simulink model "StateError"  (R2017b)
settings: Solver=FixedStepAuto  StartTime=0.0  StopTime=10.0  FixedStep=0.08  RelTol=1e-3
settings Model: Creator=hbourbou  LastModifiedBy=hbourbou

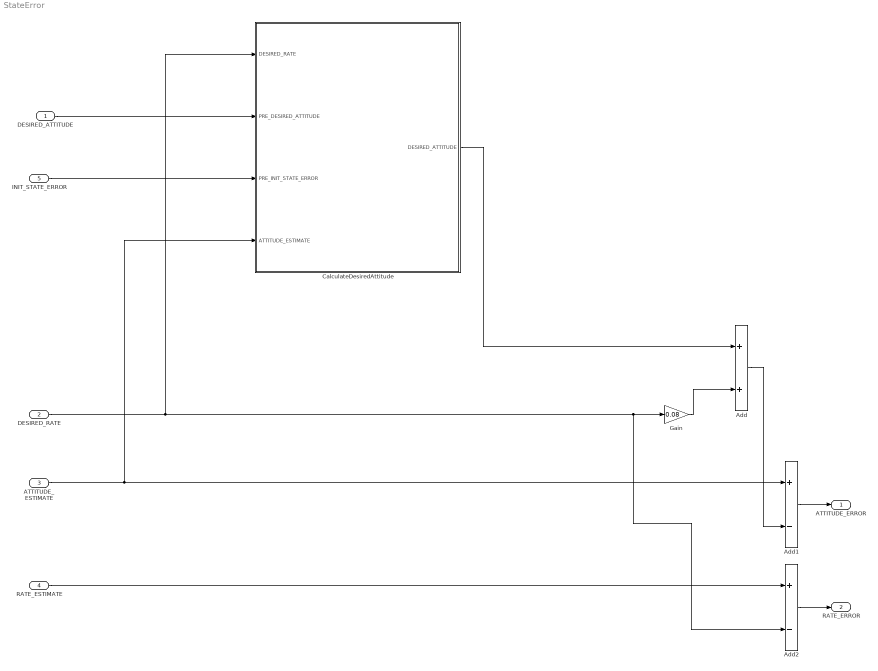
== system StateError ==
  DESIRED_ATTITUDE : Inport  PortDimensions=3
  DESIRED_RATE : Inport  Port=2  PortDimensions=3
  ATTITUDE_ESTIMATE : Inport  Port=3  PortDimensions=3
  RATE_ESTIMATE : Inport  Port=4  PortDimensions=3
  INIT_STATE_ERROR : Inport  Port=5
  Add : Sum
  Add1 : Sum  Inputs=+-
  Add2 : Sum  Inputs=+-
  CalculateDesiredAttitude : Subsystem
  Gain : Gain  Gain=0.08
  ATTITUDE_ERROR : Outport
  RATE_ERROR : Outport  Port=2
  wires:
  RATE_ESTIMATE/1 -> Add2/1
  Add/1 -> Add1/2
  Gain/1 -> Add/2
  Add1/1 -> ATTITUDE_ERROR/1
  CalculateDesiredAttitude/1(DESIRED_ATTITUDE) -> Add/1
  Add2/1 -> RATE_ERROR/1
  ATTITUDE_ESTIMATE/1 -> CalculateDesiredAttitude/4(ATTITUDE_ESTIMATE), Add1/1
  INIT_STATE_ERROR/1 -> CalculateDesiredAttitude/3(PRE_INIT_STATE_ERROR)
  DESIRED_RATE/1 -> CalculateDesiredAttitude/1(DESIRED_RATE), Add2/2, Gain/1
  DESIRED_ATTITUDE/1 -> CalculateDesiredAttitude/2(PRE_DESIRED_ATTITUDE)

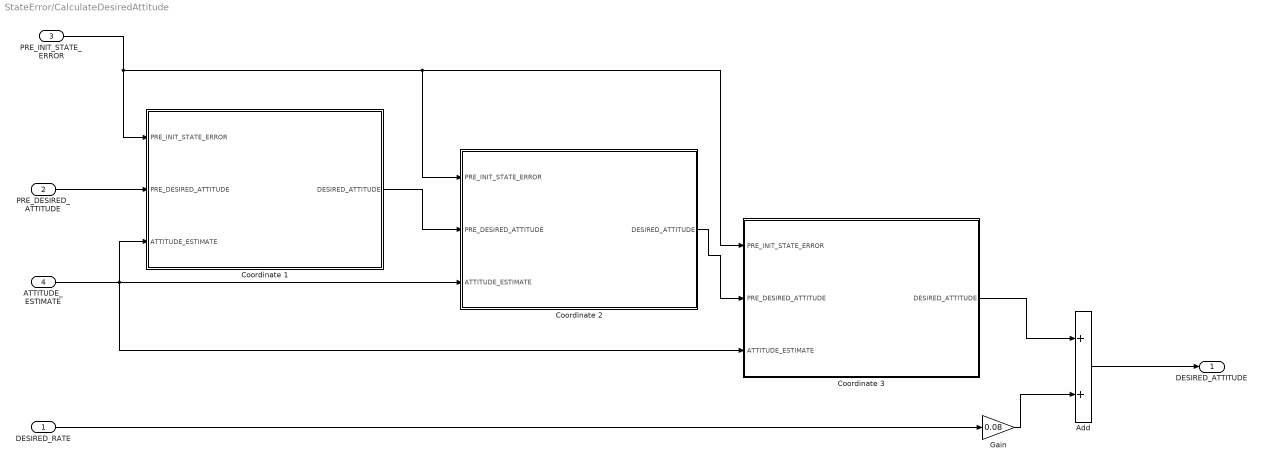
== system StateError/CalculateDesiredAttitude ==
  DESIRED_RATE : Inport  PortDimensions=3
  PRE_DESIRED_ATTITUDE : Inport  Port=2  PortDimensions=3
  PRE_INIT_STATE_ERROR : Inport  Port=3  OutDataTypeStr=boolean  PortDimensions=3
  ATTITUDE_ESTIMATE : Inport  Port=4  PortDimensions=3
  Add : Sum
  Coordinate 1 : Subsystem
  Coordinate 2 : Subsystem
  Coordinate 3 : Subsystem
  Gain : Gain  Gain=0.08
  DESIRED_ATTITUDE : Outport
  wires:
  PRE_INIT_STATE_ERROR/1 -> Coordinate 3/1(PRE_INIT_STATE_ERROR), Coordinate 2/1(PRE_INIT_STATE_ERROR), Coordinate 1/1(PRE_INIT_STATE_ERROR)
  PRE_DESIRED_ATTITUDE/1 -> Coordinate 1/2(PRE_DESIRED_ATTITUDE)
  ATTITUDE_ESTIMATE/1 -> Coordinate 2/3(ATTITUDE_ESTIMATE), Coordinate 3/3(ATTITUDE_ESTIMATE), Coordinate 1/3(ATTITUDE_ESTIMATE)
  Add/1 -> DESIRED_ATTITUDE/1
  Coordinate 3/1(DESIRED_ATTITUDE) -> Add/1
  Coordinate 1/1(DESIRED_ATTITUDE) -> Coordinate 2/2(PRE_DESIRED_ATTITUDE)
  DESIRED_RATE/1 -> Gain/1
  Gain/1 -> Add/2
  Coordinate 2/1(DESIRED_ATTITUDE) -> Coordinate 3/2(PRE_DESIRED_ATTITUDE)

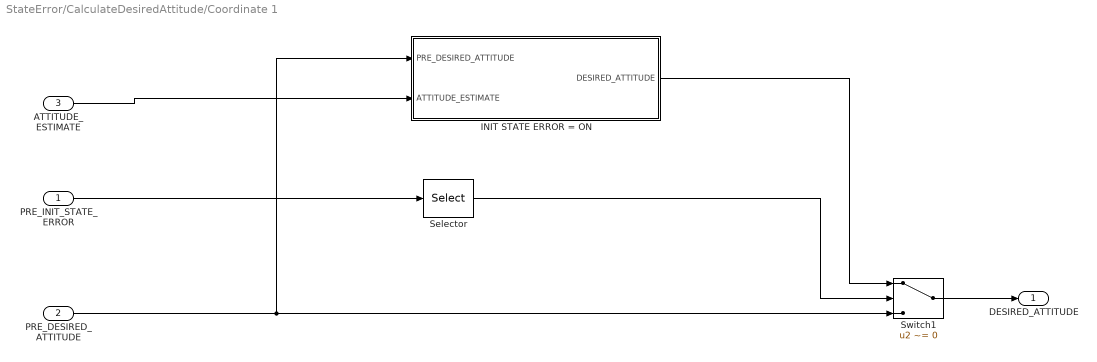
== system StateError/CalculateDesiredAttitude/Coordinate 1 ==
  PRE_INIT_STATE_ERROR : Inport
  PRE_DESIRED_ATTITUDE : Inport  Port=2
  ATTITUDE_ESTIMATE : Inport  Port=3
  INIT STATE ERROR = ON : Subsystem  TreatAsAtomicUnit=on
  Selector : Selector  InputPortWidth=3  IndexOptions=Index vector (dialog)  Indices=[1]  OutputSizes=1
  Switch1 : Switch  Criteria=u2 ~= 0
  DESIRED_ATTITUDE : Outport
  wires:
  PRE_INIT_STATE_ERROR/1 -> Selector/1
  Switch1/1 -> DESIRED_ATTITUDE/1
  INIT STATE ERROR = ON/1(DESIRED_ATTITUDE) -> Switch1/1
  PRE_DESIRED_ATTITUDE/1 -> INIT STATE ERROR = ON/1(PRE_DESIRED_ATTITUDE), Switch1/3
  ATTITUDE_ESTIMATE/1 -> INIT STATE ERROR = ON/2(ATTITUDE_ESTIMATE)
  Selector/1 -> Switch1/2

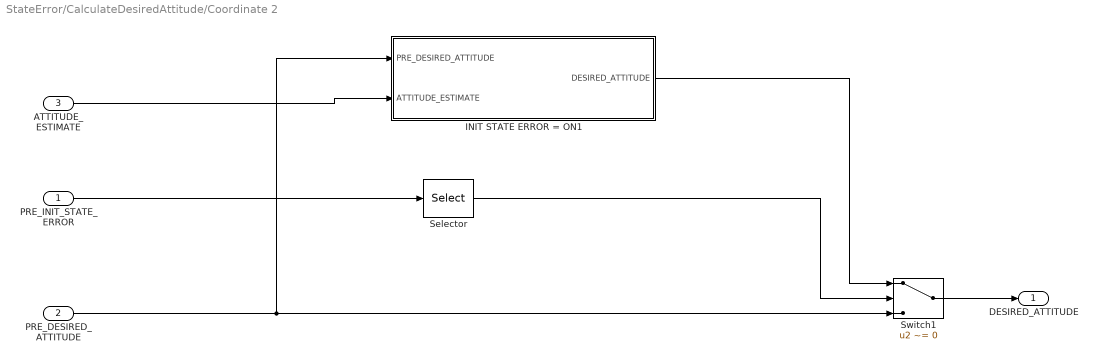
== system StateError/CalculateDesiredAttitude/Coordinate 2 ==
  PRE_INIT_STATE_ERROR : Inport
  PRE_DESIRED_ATTITUDE : Inport  Port=2
  ATTITUDE_ESTIMATE : Inport  Port=3
  INIT STATE ERROR = ON1 : Subsystem  TreatAsAtomicUnit=on
  Selector : Selector  InputPortWidth=3  IndexOptions=Index vector (dialog)  Indices=2  OutputSizes=1
  Switch1 : Switch  Criteria=u2 ~= 0
  DESIRED_ATTITUDE : Outport
  wires:
  PRE_INIT_STATE_ERROR/1 -> Selector/1
  Switch1/1 -> DESIRED_ATTITUDE/1
  INIT STATE ERROR = ON1/1(DESIRED_ATTITUDE) -> Switch1/1
  PRE_DESIRED_ATTITUDE/1 -> INIT STATE ERROR = ON1/1(PRE_DESIRED_ATTITUDE), Switch1/3
  ATTITUDE_ESTIMATE/1 -> INIT STATE ERROR = ON1/2(ATTITUDE_ESTIMATE)
  Selector/1 -> Switch1/2

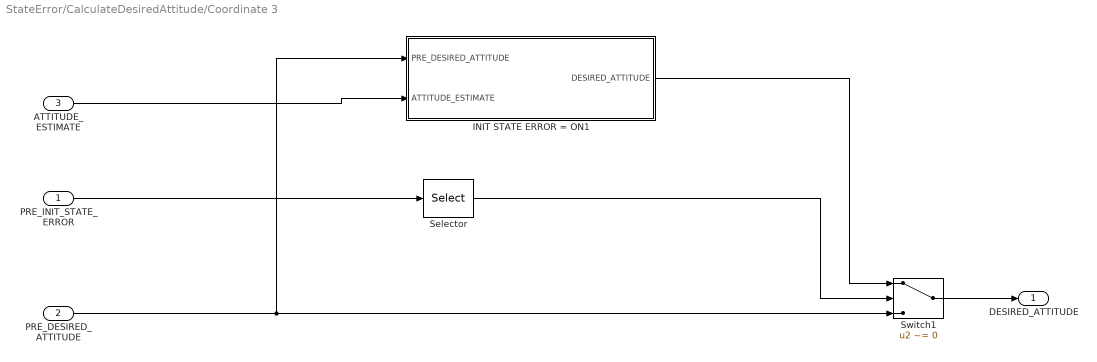
== system StateError/CalculateDesiredAttitude/Coordinate 3 ==
  PRE_INIT_STATE_ERROR : Inport
  PRE_DESIRED_ATTITUDE : Inport  Port=2
  ATTITUDE_ESTIMATE : Inport  Port=3
  INIT STATE ERROR = ON1 : Subsystem  TreatAsAtomicUnit=on
  Selector : Selector  InputPortWidth=3  IndexOptions=Index vector (dialog)  Indices=3  OutputSizes=1
  Switch1 : Switch  Criteria=u2 ~= 0
  DESIRED_ATTITUDE : Outport
  wires:
  PRE_INIT_STATE_ERROR/1 -> Selector/1
  Switch1/1 -> DESIRED_ATTITUDE/1
  INIT STATE ERROR = ON1/1(DESIRED_ATTITUDE) -> Switch1/1
  PRE_DESIRED_ATTITUDE/1 -> INIT STATE ERROR = ON1/1(PRE_DESIRED_ATTITUDE), Switch1/3
  ATTITUDE_ESTIMATE/1 -> INIT STATE ERROR = ON1/2(ATTITUDE_ESTIMATE)
  Selector/1 -> Switch1/2

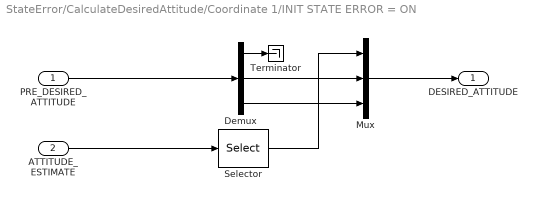
== system StateError/CalculateDesiredAttitude/Coordinate 1/INIT STATE ERROR = ON ==
  PRE_DESIRED_ATTITUDE : Inport
  ATTITUDE_ESTIMATE : Inport  Port=2
  Demux : Demux  Outputs=3
  Mux : Mux  Inputs=3
  Selector : Selector  InputPortWidth=3  IndexOptions=Index vector (dialog)  Indices=[1]  OutputSizes=1
  Terminator : Terminator
  DESIRED_ATTITUDE : Outport
  wires:
  PRE_DESIRED_ATTITUDE/1 -> Demux/1
  Selector/1 -> Mux/1
  Demux/2 -> Mux/2
  Demux/3 -> Mux/3
  Mux/1 -> DESIRED_ATTITUDE/1
  Demux/1 -> Terminator/1
  ATTITUDE_ESTIMATE/1 -> Selector/1

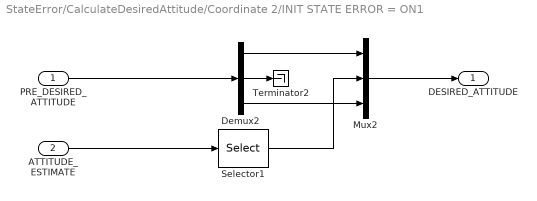
== system StateError/CalculateDesiredAttitude/Coordinate 2/INIT STATE ERROR = ON1 ==
  PRE_DESIRED_ATTITUDE : Inport
  ATTITUDE_ESTIMATE : Inport  Port=2
  Demux2 : Demux  Outputs=3
  Mux2 : Mux  Inputs=3
  Selector1 : Selector  InputPortWidth=3  IndexOptions=Index vector (dialog)  Indices=2  OutputSizes=1
  Terminator2 : Terminator
  DESIRED_ATTITUDE : Outport
  wires:
  Demux2/3 -> Mux2/3
  ATTITUDE_ESTIMATE/1 -> Selector1/1
  Mux2/1 -> DESIRED_ATTITUDE/1
  PRE_DESIRED_ATTITUDE/1 -> Demux2/1
  Demux2/2 -> Terminator2/1
  Demux2/1 -> Mux2/1
  Selector1/1 -> Mux2/2

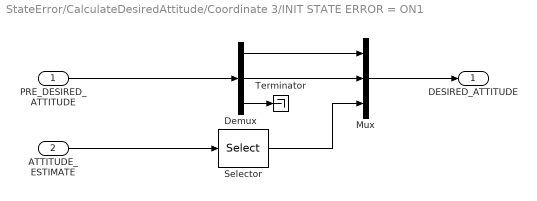
== system StateError/CalculateDesiredAttitude/Coordinate 3/INIT STATE ERROR = ON1 ==
  PRE_DESIRED_ATTITUDE : Inport
  ATTITUDE_ESTIMATE : Inport  Port=2
  Demux : Demux  Outputs=3
  Mux : Mux  Inputs=3
  Selector : Selector  InputPortWidth=3  IndexOptions=Index vector (dialog)  Indices=3  OutputSizes=1
  Terminator : Terminator
  DESIRED_ATTITUDE : Outport
  wires:
  PRE_DESIRED_ATTITUDE/1 -> Demux/1
  ATTITUDE_ESTIMATE/1 -> Selector/1
  Demux/2 -> Mux/2
  Mux/1 -> DESIRED_ATTITUDE/1
  Demux/3 -> Terminator/1
  Selector/1 -> Mux/3
  Demux/1 -> Mux/1
